simulink model "Torque_controller_using_LIM_wo_simulink"  (R2018a)
settings: Solver=VariableStepAuto  StartTime=0.0  StopTime=2  RelTol=1e-3
values from neighbouring files (symbols this model uses):
  fn = 100    [LIM_thrust_controller_parameters.m]    (also in lim_model_pu.m = 70)
  Ibase = Pn/(1.5*Vbase)    [LIM_thrust_controller_parameters.m]    (also in lim_model_pu.m)
  Imax = 4*Ibase    [LIM_thrust_controller_parameters.m]
  Imin = 0.1*Inom    (= 2.76073619632)    [LIM_thrust_controller_parameters.m]
  Inom = psi_ref/LM    (= 27.6073619632)    [LIM_thrust_controller_parameters.m]
  ki = ac^2*Lo    [LIM_thrust_controller_parameters.m]
  kp = ac*Lo    [LIM_thrust_controller_parameters.m]
  Lm = 32.6e-3    (= 0.0326)    [LIM_thrust_controller_parameters.m]    (also in lim_model.m; lim_model_pu.m = 32.6e-3/L_base)
  Lo = Ls    (= 0.0401)    [LIM_thrust_controller_parameters.m]
  Lr = 33.1e-3    (= 0.0331)    [LIM_thrust_controller_parameters.m]    (also in lim_model.m; lim_model_pu.m = 33.1e-3/L_base)
  p = 4    [LIM_thrust_controller_parameters.m]    (also in lim_model.m; lim_model_pu.m)
  Ra = ac*Lo - RR    [LIM_thrust_controller_parameters.m]
  RR = 2.7    [LIM_thrust_controller_parameters.m]
  tau = 0.2    [LIM_thrust_controller_parameters.m]    (also in lim_model.m = 0.066; lim_model_pu.m)
  Ts = 5e-6    (= 5e-06)    [LIM_thrust_controller_parameters.m]
  Tsc = 1/(fsw*50)    (= 1e-05)    [LIM_thrust_controller_parameters.m]
  Ty = Lr/RR    (= 0.0122592592593)    [LIM_thrust_controller_parameters.m]
  Vbase = Vn/sqrt(3)*sqrt(2)    [LIM_thrust_controller_parameters.m]    (also in lim_model_pu.m)
  w1 = 1    [LIM_thrust_controller_parameters.m]
  wbase = 2*pi*fn    (= 628.318530718)    [LIM_thrust_controller_parameters.m]    (also in lim_model_pu.m = 439.822971503)
  xi = (Lo+LM)/Lo    (= 1.81296758105)    [LIM_thrust_controller_parameters.m]
undefined symbols (not defined in the file or in its folder): DiscIntNeverNeededParam, id_ref, sigbuilder_block
libraries: powerlib_meascontrol x5, simulink x1
settings Model: Creator=akashsin  LastModifiedBy=akashsin

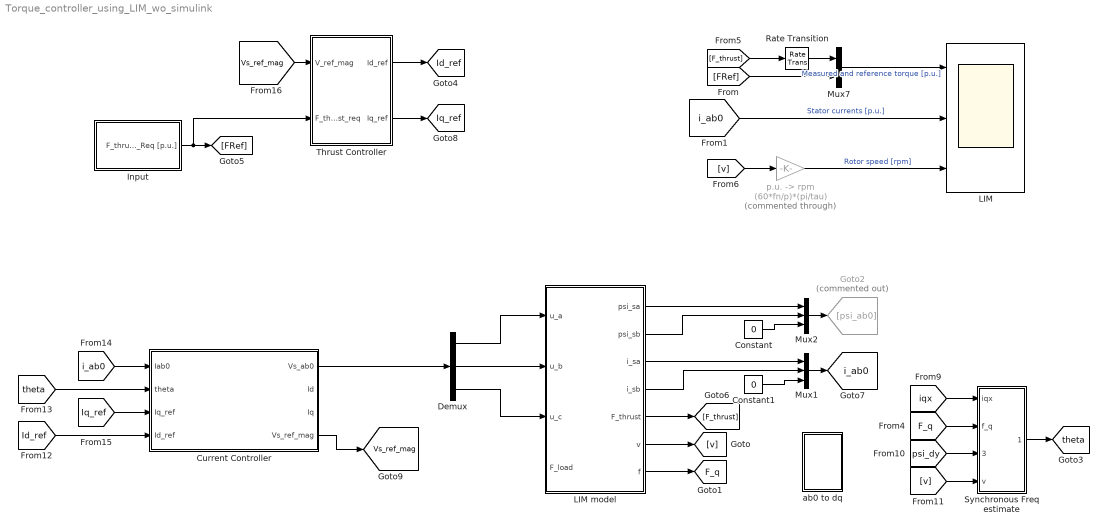
== system Torque_controller_using_LIM_wo_simulink ==
  Constant : Constant  Value=0  SampleTime=Tsc
  Constant1 : Constant  Value=0  SampleTime=Tsc
  Current Controller : Subsystem
  Demux : Demux  Outputs=3
  Goto2 : Goto  Commented=on  GotoTag=psi_ab0
  Input : Subsystem  Tag=STV Subsys  LoadFcn=sigbuilder_block('load');  StartFcn=sigbuilder_block('start');  StopFcn=sigbuilder_block('stop');  ClipboardFcn=sigbuilder_block('clipboard');  mask(Sigbuilder block){tuvar=[0:10]}
      mask help: Simulink:masks:SigbuilderBlock_MD
      mask init:
      | if ~strcmp(get_param(bdroot(gcbh),'SimulationStatus'),'stopped') tuvar = sigbuilder_block('maskInit'); end
      settings: CopyFcn=sigbuilder_block('copy');  DeleteFcn=sigbuilder_block('delete');  ModelCloseFcn=sigbuilder_block('modelClose');  PreSaveFcn=sigbuilder_block('preSave');  PauseFcn=sigbuilder_block('pause');  ContinueFcn=sigbuilder_block('continue');  NameChangeFcn=sigbuilder_block('namechange');  OpenFcn=sigbuilder_block('open',[683.25 241.5 615.75 445.5 ]);  CloseFcn=sigbuilder_block('close');
      mask Display: plot(0, 0, 100, 100,[2, 2, 32, 32, 2], [68, 8, 8, 68, 68],[32, 2], [38, 38], [32, 19, 2],[53, 60, 44], [32, 17, 17, 2],[16, 16, 31, 31]);txt = getActiveGroup(gcbh);text(2, 100, txt,'verticalAlignment', 'top');
  LIM : Scope  NumInputPorts=3
  LIM model : Subsystem
  Mux1 : Mux  Inputs=3
  Mux2 : Mux  Inputs=3
  Mux7 : Mux  Inputs=2
  Rate Transition : RateTransition  OutPortSampleTime=Tsc
  Synchronous Freq estimate : Subsystem
  Thrust Controller : Subsystem
  ab0 to dq : Subsystem
  "p.u. -> rpm" : Gain  Commented=through  Gain=(60*fn/p)*(pi/tau)
  tag scope: F_q=global, Id_ref=global, Iq_ref=global, Vs_ref_mag=global, i_ab0=global, theta=global
  wires:
  Thrust Controller/2(Iq_ref) -> [Iq_ref]
  Thrust Controller/1(Id_ref) -> [Id_ref]
  Input/1(F_thrust_Req [p.u.]) -> [FRef], Thrust Controller/2(F_thrust_req)
  [Vs_ref_mag] -> Thrust Controller/1(V_ref_mag)
  Synchronous Freq estimate/1(theta) -> [theta]
  [v] -> Synchronous Freq estimate/4(v)
  [psi_dy] -> Synchronous Freq estimate/3(psi_dy)
  [F_q] -> Synchronous Freq estimate/2(f_q)
  [iqx] -> Synchronous Freq estimate/1(iqx)
  Mux1/1 -> [i_ab0]
  LIM model/5(F_thrust) -> [F_thrust]
  Constant1/1 -> Mux1/3
  LIM model/4(i_sb) -> Mux1/2
  LIM model/3(i_sa) -> Mux1/1
  Mux2/1 -> Goto2/1
  Constant/1 -> Mux2/3
  LIM model/2(psi_sb) -> Mux2/2
  LIM model/1(psi_sa) -> Mux2/1
  LIM model/6(v) -> [v]
  LIM model/7(f) -> [F_q]
  Demux/3 -> LIM model/3(u_c)
  Demux/1 -> LIM model/1(u_a)
  Demux/2 -> LIM model/2(u_b)
  [FRef] -> Mux7/2
  [v] -> "p.u. -> rpm"/1
  "p.u. -> rpm"/1 -> LIM/3  "Rotor speed [rpm]"
  Mux7/1 -> LIM/1  "Measured and reference torque [p.u.]"
  Rate Transition/1 -> Mux7/1
  [F_thrust] -> Rate Transition/1
  [i_ab0] -> LIM/2  "Stator currents [p.u.]"
  Current Controller/4(Vs_ref_mag) -> [Vs_ref_mag]
  Current Controller/1(Vs_ab0) -> Demux/1
  [Id_ref] -> Current Controller/4(Id_ref)
  [Iq_ref] -> Current Controller/3(Iq_ref)
  [theta] -> Current Controller/2(theta)
  [i_ab0] -> Current Controller/1(Iab0)

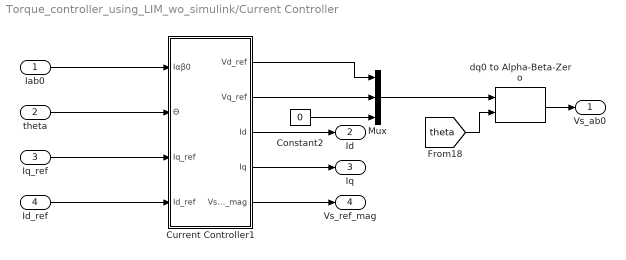
== system Torque_controller_using_LIM_wo_simulink/Current Controller ==
  Iab0 : Inport
  theta : Inport  Port=2
  Iq_ref : Inport  Port=3
  Id_ref : Inport  Port=4
  Constant2 : Constant  Value=0  SampleTime=Tsc
  Current Controller1 : Subsystem
  Mux : Mux  Inputs=3
  dq0 to Alpha-Beta-Zero : powerlib_meascontrol/Transformations/dq0 to Alpha-Beta-Zero  Alignment=Aligned with phase A axis
      settings: SourceProductName=Simscape Power Systems  SourceProductBaseCode=PS
  Vs_ab0 : Outport
  Id : Outport  Port=2
  Iq : Outport  Port=3
  Vs_ref_mag : Outport  Port=4
  wires:
  Current Controller1/5(Vs_ref_mag) -> Vs_ref_mag/1
  Id_ref/1 -> Current Controller1/4(Id_ref)
  Iab0/1 -> Current Controller1/1(Iαβ0)
  theta/1 -> Current Controller1/2(Θ)
  Iq_ref/1 -> Current Controller1/3(Iq_ref)
  Current Controller1/4(Iq) -> Iq/1
  [theta] -> dq0 to Alpha-Beta-Zero/2
  Mux/1 -> dq0 to Alpha-Beta-Zero/1
  dq0 to Alpha-Beta-Zero/1 -> Vs_ab0/1
  Current Controller1/3(Id) -> Id/1
  Constant2/1 -> Mux/3
  Current Controller1/2(Vq_ref) -> Mux/2
  Current Controller1/1(Vd_ref) -> Mux/1

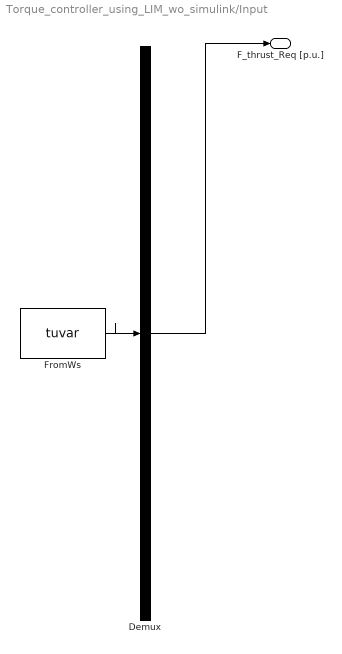
== system Torque_controller_using_LIM_wo_simulink/Input ==
  Demux : Demux  Tag=STV Demux  Outputs=1
  FromWs : FromWorkspace  Tag=STV FromWs  VariableName=tuvar  SampleTime=0
      SigBuilderData=|
      | common.afterFinalStr = 'Extrapolate'
      | common.sampleTime = 0
      | dataSet.timeRange = [0 2]
      | dataSet.name = 'Test 1'
      | sbobj.Groups.Name = 'Test 1'
      | sbobj.Groups.Signals.Name = 'F_thrust_Req [p.u.]'
      | sbobj.Groups.Signals.XData = [0 0.1 0.1 1.07 1.345 1.345 1.6 1.6 2]
      | sbobj.Groups.Signals.YData = [0 0 1.005 1.005 1.005 0.75 0.745 -0.005 -0.005]
      | sbobj.Groups.TimeRange = [0 2]
  F_thrust_Req [p.u.] : Outport  Tag=STV Outport
  wires:
  FromWs/1 -> Demux/1
  Demux/1 -> F_thrust_Req [p.u.]/1

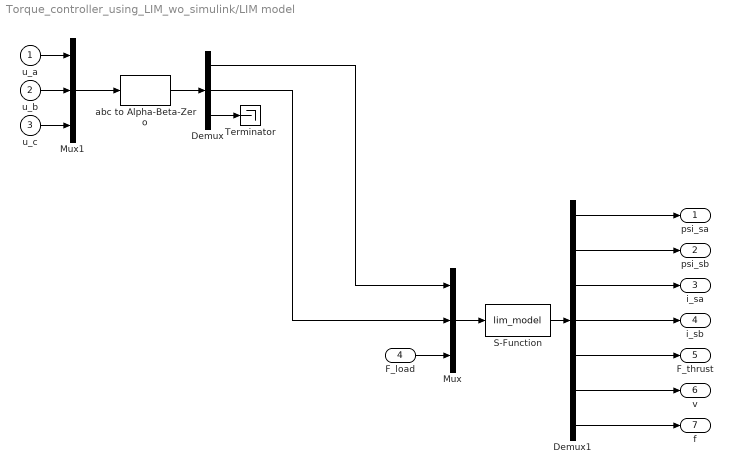
== system Torque_controller_using_LIM_wo_simulink/LIM model ==
  u_a : Inport
  u_b : Inport  Port=2
  u_c : Inport  Port=3
  F_load : Inport  Port=4
  Demux : Demux  Outputs=3
  Demux1 : Demux  Outputs=7
  Mux : Mux  Inputs=3
  Mux1 : Mux  Inputs=3
  S-Function : S-Function  FunctionName=lim_model  SFunctionDeploymentMode=off  EnableBusSupport=off
  Terminator : Terminator
  abc to Alpha-Beta-Zero : powerlib_meascontrol/Transformations/abc to Alpha-Beta-Zero
      settings: SourceProductName=Simscape Power Systems
  psi_sa : Outport
  psi_sb : Outport  Port=2
  i_sa : Outport  Port=3
  i_sb : Outport  Port=4
  F_thrust : Outport  Port=5
  v : Outport  Port=6
  f : Outport  Port=7
  wires:
  F_load/1 -> Mux/3
  Mux/1 -> S-Function/1
  Demux1/2 -> psi_sb/1
  Demux1/3 -> i_sa/1
  S-Function/1 -> Demux1/1
  Demux1/7 -> f/1
  Demux/1 -> Mux/1
  Demux1/4 -> i_sb/1
  Demux1/6 -> v/1
  Demux1/1 -> psi_sa/1
  Demux/2 -> Mux/2
  Demux1/5 -> F_thrust/1
  u_a/1 -> Mux1/1
  Demux/3 -> Terminator/1
  u_c/1 -> Mux1/3
  u_b/1 -> Mux1/2
  abc to Alpha-Beta-Zero/1 -> Demux/1
  Mux1/1 -> abc to Alpha-Beta-Zero/1

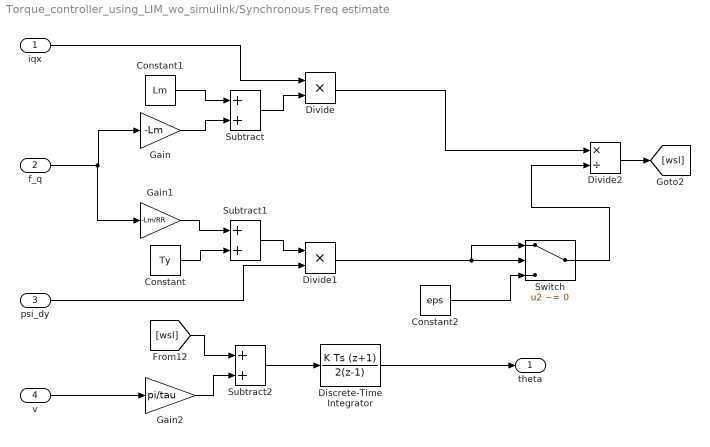
== system Torque_controller_using_LIM_wo_simulink/Synchronous Freq estimate ==
  iqx : Inport
  f_q : Inport  Port=2
  psi_dy : Inport  Port=3
  v : Inport  Port=4
  Constant : Constant  Value=Ty  SampleTime=Tsc
  Constant1 : Constant  Value=Lm  SampleTime=Tsc
  Constant2 : Constant  Value=eps  SampleTime=Tsc
  Discrete-Time Integrator : DiscreteIntegrator  IntegratorMethod=Integration: Trapezoidal  SampleTime=Tsc  ICPrevOutput=DiscIntNeverNeededParam  ICPrevScaledInput=DiscIntNeverNeededParam
  Divide : Product  Inputs=**
  Divide1 : Product  Inputs=**
  Divide2 : Product  Inputs=*/
  Gain : Gain  Gain=-Lm
  Gain1 : Gain  Gain=-Lm/RR
  Gain2 : Gain  Gain=pi/tau
  Subtract : Sum
  Subtract1 : Sum
  Subtract2 : Sum
  Switch : Switch  Criteria=u2 ~= 0
  theta : Outport
  wires:
  Divide2/1 -> [wsl]
  Switch/1 -> Divide2/2
  Constant2/1 -> Switch/3
  Divide1/1 -> Switch/2, Switch/1
  iqx/1 -> Divide/1
  v/1 -> Gain2/1
  Gain2/1 -> Subtract2/2
  Gain1/1 -> Subtract1/1
  Constant/1 -> Subtract1/2
  [wsl] -> Subtract2/1
  Divide/1 -> Divide2/1
  psi_dy/1 -> Divide1/2
  Subtract1/1 -> Divide1/1
  Gain/1 -> Subtract/2
  f_q/1 -> Gain/1, Gain1/1
  Discrete-Time Integrator/1 -> theta/1
  Subtract2/1 -> Discrete-Time Integrator/1
  Subtract/1 -> Divide/2
  Constant1/1 -> Subtract/1

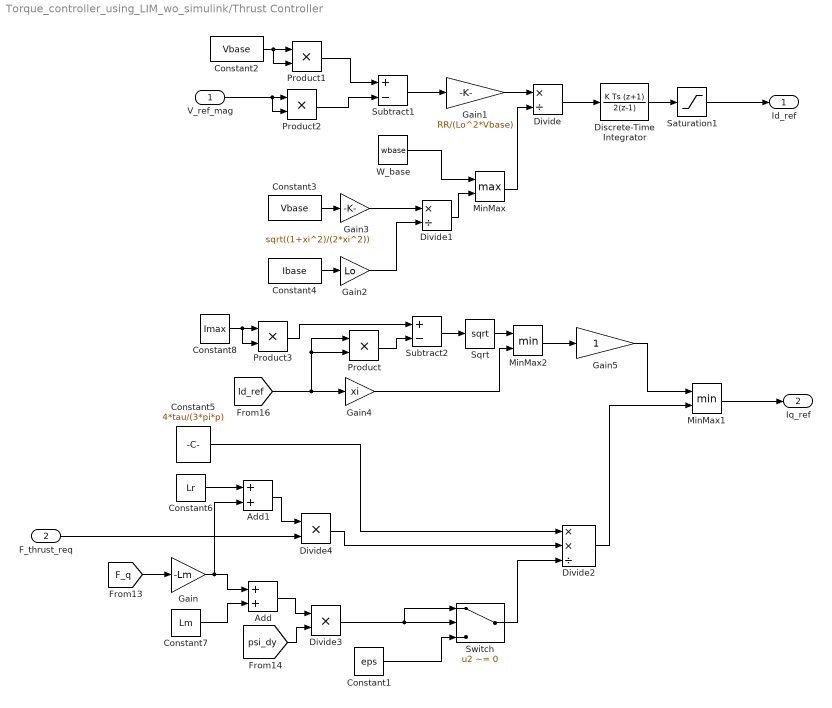
== system Torque_controller_using_LIM_wo_simulink/Thrust Controller ==
  V_ref_mag : Inport
  F_thrust_req : Inport  Port=2
  Add : Sum
  Add1 : Sum
  Constant1 : Constant  Value=eps  SampleTime=Tsc
  Constant2 : Constant  Value=Vbase  SampleTime=Tsc
  Constant3 : Constant  Value=Vbase  SampleTime=Tsc
  Constant4 : Constant  Value=Ibase  SampleTime=Tsc
  Constant5 : Constant  Value=4*tau/(3*pi*p)  SampleTime=Tsc
  Constant6 : Constant  Value=Lr  SampleTime=Tsc
  Constant7 : Constant  Value=Lm  SampleTime=Tsc
  Constant8 : Constant  Value=Imax  SampleTime=Tsc
  Discrete-Time Integrator : DiscreteIntegrator  IntegratorMethod=Integration: Trapezoidal  SampleTime=Ts  ICPrevOutput=DiscIntNeverNeededParam  ICPrevScaledInput=DiscIntNeverNeededParam
  Divide : Product  Inputs=*/
  Divide1 : Product  Inputs=*/
  Divide2 : Product  Inputs=**/
  Divide3 : Product  Inputs=**
  Divide4 : Product  Inputs=**
  Gain : Gain  Gain=-Lm
  Gain1 : Gain  Gain=RR/(Lo^2*Vbase)
  Gain2 : Gain  Gain=Lo
  Gain3 : Gain  Gain=sqrt((1+xi^2)/(2*xi^2))
  Gain4 : Gain  Gain=xi
  Gain5 : Gain
  MinMax : MinMax  Function=max  Inputs=2
  MinMax1 : MinMax  Inputs=2
  MinMax2 : MinMax  Inputs=2
  Product{,1..3} (4 alike) : Product
  Saturation1 : Saturate  UpperLimit=Inom  LowerLimit=Imin
  Sqrt : Sqrt  SaturateOnIntegerOverflow=on
  Subtract1 : Sum  Inputs=+-
  Subtract2 : Sum  Inputs=+-
  Switch : Switch  Criteria=u2 ~= 0
  W_base : Constant  Value=wbase  SampleTime=Tsc
  Id_ref : Outport
  Iq_ref : Outport  Port=2
  wires:
  Switch/1 -> Divide2/3
  Constant1/1 -> Switch/3
  Divide3/1 -> Switch/2, Switch/1
  Gain2/1 -> Divide1/2
  Product1/1 -> Subtract1/1
  Constant3/1 -> Gain3/1
  Gain5/1 -> MinMax1/1
  Gain1/1 -> Divide/1
  Subtract1/1 -> Gain1/1
  MinMax2/1 -> Gain5/1
  V_ref_mag/1 -> Product2/1, Product2/2
  Subtract2/1 -> Sqrt/1
  Product3/1 -> Subtract2/1
  Divide1/1 -> MinMax/2
  Gain4/1 -> MinMax2/2
  MinMax1/1 -> Iq_ref/1
  Constant4/1 -> Gain2/1
  Sqrt/1 -> MinMax2/1
  Product/1 -> Subtract2/2
  Constant8/1 -> Product3/1, Product3/2
  Constant5/1 -> Divide2/1
  Divide/1 -> Discrete-Time Integrator/1
  MinMax/1 -> Divide/2
  Discrete-Time Integrator/1 -> Saturation1/1
  Product2/1 -> Subtract1/2
  Constant6/1 -> Add1/1
  [Id_ref] -> Gain4/1, Product/1, Product/2
  [psi_dy] -> Divide3/2
  Divide2/1 -> MinMax1/2
  Add/1 -> Divide3/1
  Add1/1 -> Divide4/1
  [F_q] -> Gain/1
  W_base/1 -> MinMax/1
  Saturation1/1 -> Id_ref/1
  Constant7/1 -> Add/2
  Constant2/1 -> Product1/1, Product1/2
  Gain3/1 -> Divide1/1
  Divide4/1 -> Divide2/2
  Gain/1 -> Add/1, Add1/2
  F_thrust_req/1 -> Divide4/2

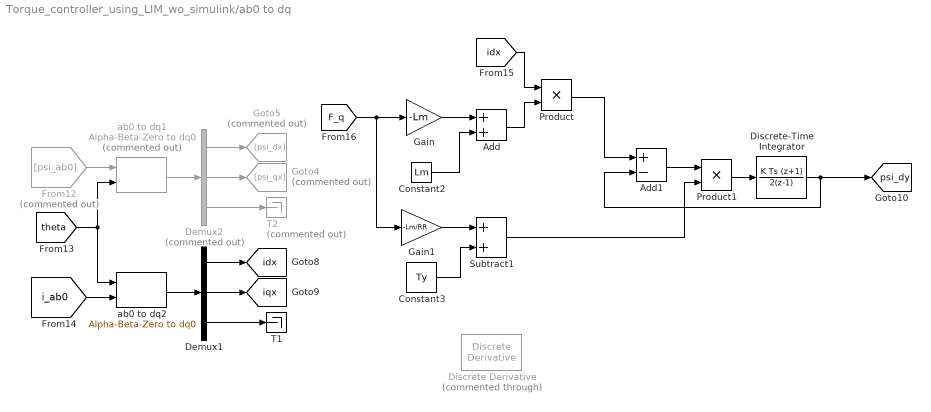
== system Torque_controller_using_LIM_wo_simulink/ab0 to dq ==
  Add : Sum
  Add1 : Sum  Inputs=+-
  Constant2 : Constant  Value=Lm  SampleTime=Tsc
  Constant3 : Constant  Value=Ty  SampleTime=Tsc
  Demux1 : Demux  Outputs=3
  Demux2 : Demux  Commented=on  Outputs=3
  Discrete Derivative : simulink/Quick Insert/Discrete/Discrete Derivative  Commented=through  gainval=1.0  ICPrevScaledInput=0.0  OutMin=[]  OutMax=[]  OutDataType=fixdt(1, 16)  OutScaling=2^-10  DoSatur=off
      settings: SourceProductName=Simulink  SourceProductBaseCode=SL
  Discrete-Time Integrator : DiscreteIntegrator  IntegratorMethod=Integration: Trapezoidal  SampleTime=Tsc  ICPrevOutput=DiscIntNeverNeededParam  ICPrevScaledInput=DiscIntNeverNeededParam
  From12 : From  Commented=on  GotoTag=psi_ab0
  Gain : Gain  Gain=-Lm
  Gain1 : Gain  Gain=-Lm/RR
  Goto4 : Goto  Commented=on  GotoTag=psi_qx
  Goto5 : Goto  Commented=on  GotoTag=psi_dx
  Product : Product
  Product1 : Product
  Subtract1 : Sum
  T1 : Terminator
  T2 : Terminator  Commented=on
  ab0 to dq1 : powerlib_meascontrol/Transformations/Alpha-Beta-Zero to dq0  Commented=on  Alignment=Aligned with phase A axis
      settings: SourceProductName=Simscape Power Systems
  ab0 to dq2 : powerlib_meascontrol/Transformations/Alpha-Beta-Zero to dq0  Alignment=Aligned with phase A axis
      settings: SourceProductName=Simscape Power Systems
  tag scope: idx=global, iqx=global, psi_dy=global
  wires:
  Add/1 -> Product/2
  Discrete-Time Integrator/1 -> Add1/2, [psi_dy]
  Product1/1 -> Discrete-Time Integrator/1
  Subtract1/1 -> Product1/2
  Add1/1 -> Product1/1
  Demux1/1 -> [idx]
  Gain1/1 -> Subtract1/1
  Product/1 -> Add1/1
  [i_ab0] -> ab0 to dq2/1
  Constant2/1 -> Add/2
  Demux2/1 -> Goto5/1
  ab0 to dq1/1 -> Demux2/1
  Demux2/2 -> Goto4/1
  From12/1 -> ab0 to dq1/1
  Demux1/2 -> [iqx]
  Gain/1 -> Add/1
  Demux1/3 -> T1/1
  ab0 to dq2/1 -> Demux1/1
  [idx] -> Product/1
  Demux2/3 -> T2/1
  Constant3/1 -> Subtract1/2
  [theta] -> ab0 to dq1/2, ab0 to dq2/2
  [F_q] -> Gain/1, Gain1/1

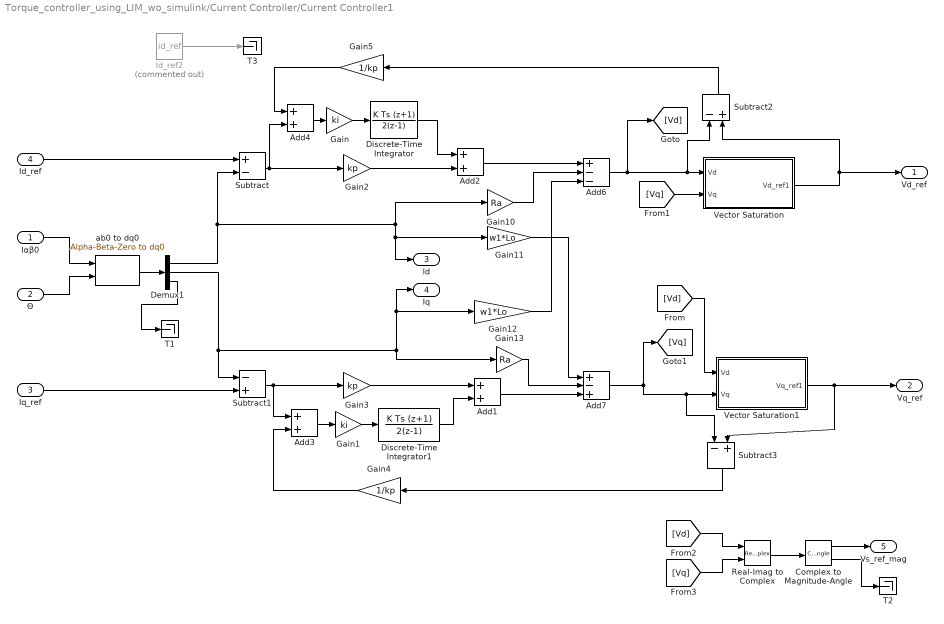
== system Torque_controller_using_LIM_wo_simulink/Current Controller/Current Controller1 ==
  Iαβ0 : Inport
  Θ : Inport  Port=2
  Iq_ref : Inport  Port=3
  Id_ref : Inport  Port=4
  Add{1..4} (4 alike) : Sum
  Add6 : Sum  Inputs=+--
  Add7 : Sum  Inputs=+-+
  Complex to Magnitude-Angle : ComplexToMagnitudeAngle
  Demux1 : Demux  Outputs=3
  Discrete-Time Integrator : DiscreteIntegrator  IntegratorMethod=Integration: Trapezoidal  SampleTime=Ts  ICPrevOutput=DiscIntNeverNeededParam  ICPrevScaledInput=DiscIntNeverNeededParam
  Discrete-Time Integrator1 : DiscreteIntegrator  IntegratorMethod=Integration: Trapezoidal  SampleTime=Ts  ICPrevOutput=DiscIntNeverNeededParam  ICPrevScaledInput=DiscIntNeverNeededParam
  Gain : Gain  Gain=ki
  Gain1 : Gain  Gain=ki
  Gain10 : Gain  Gain=Ra
  Gain11 : Gain  Gain=w1*Lo
  Gain12 : Gain  Gain=w1*Lo
  Gain13 : Gain  Gain=Ra
  Gain2 : Gain  Gain=kp
  Gain3 : Gain  Gain=kp
  Gain4 : Gain  Gain=1/kp
  Gain5 : Gain  Gain=1/kp
  Id_ref2 : Constant  Commented=on  Value=id_ref
  Real-Imag to Complex : RealImagToComplex
  Subtract : Sum  Inputs=+-
  Subtract1 : Sum  Inputs=-+
  Subtract2 : Sum  Inputs=-+
  Subtract3 : Sum  Inputs=-+
  T1 : Terminator
  T2 : Terminator
  T3 : Terminator
  Vector Saturation : Subsystem
  Vector Saturation1 : Subsystem
  ab0 to dq0 : powerlib_meascontrol/Transformations/Alpha-Beta-Zero to dq0  Alignment=Aligned with phase A axis
      settings: SourceProductName=Simscape Power Systems
  Vd_ref : Outport
  Vq_ref : Outport  Port=2
  Id : Outport  Port=3
  Iq : Outport  Port=4
  Vs_ref_mag : Outport  Port=5
  wires:
  Id_ref/1 -> Subtract/1
  [Vq] -> Real-Imag to Complex/2
  [Vd] -> Real-Imag to Complex/1
  Id_ref2/1 -> T3/1
  Complex to Magnitude-Angle/2 -> T2/1
  Complex to Magnitude-Angle/1 -> Vs_ref_mag/1
  Real-Imag to Complex/1 -> Complex to Magnitude-Angle/1
  Vector Saturation/1(Vd_ref1) -> Subtract2/2, Vd_ref/1
  Vector Saturation1/1(Vq_ref1) -> Subtract3/2, Vq_ref/1
  [Vq] -> Vector Saturation/2(Vq)
  [Vd] -> Vector Saturation1/1(Vd)
  Θ/1 -> ab0 to dq0/2
  Add7/1 -> [Vq], Vector Saturation1/2(Vq), Subtract3/1
  Add6/1 -> [Vd], Vector Saturation/1(Vd), Subtract2/1
  Iq_ref/1 -> Subtract1/2
  Gain13/1 -> Add7/2
  Gain12/1 -> Add6/3
  Demux1/2 -> Subtract1/1, Gain13/1, Iq/1, Gain12/1
  Add1/1 -> Add7/3
  Add2/1 -> Add6/1
  Gain11/1 -> Add7/1
  Gain10/1 -> Add6/2
  Demux1/1 -> Subtract/2, Gain10/1, Id/1, Gain11/1
  Subtract2/1 -> Gain5/1
  Add4/1 -> Gain/1
  Subtract1/1 -> Gain3/1, Add3/1
  Gain1/1 -> Discrete-Time Integrator1/1
  Gain/1 -> Discrete-Time Integrator/1
  Subtract/1 -> Gain2/1, Add4/2
  ab0 to dq0/1 -> Demux1/1
  Demux1/3 -> T1/1
  Iαβ0/1 -> ab0 to dq0/1
  Gain5/1 -> Add4/1
  Gain2/1 -> Add2/2
  Gain4/1 -> Add3/2
  Add3/1 -> Gain1/1
  Discrete-Time Integrator/1 -> Add2/1
  Subtract3/1 -> Gain4/1
  Discrete-Time Integrator1/1 -> Add1/2
  Gain3/1 -> Add1/1

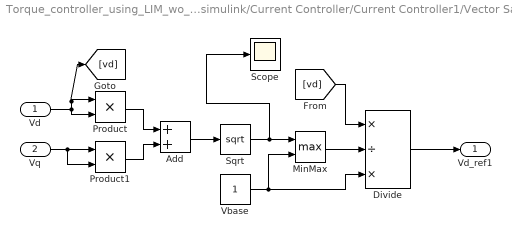
== system Torque_controller_using_LIM_wo_simulink/Current Controller/Current Controller1/Vector Saturation ==
  Vd : Inport
  Vq : Inport  Port=2
  Add : Sum
  Divide : Product  Inputs=*/*
  MinMax : MinMax  Function=max  Inputs=2
  Product : Product
  Product1 : Product
  Scope : Scope
  Sqrt : Sqrt  SaturateOnIntegerOverflow=on
  Vbase : Constant
  Vd_ref1 : Outport
  wires:
  Vbase/1 -> MinMax/2, Divide/3
  MinMax/1 -> Divide/2
  Vd/1 -> Product/2, Product/1, [vd]
  Product/1 -> Add/1
  Vq/1 -> Product1/1, Product1/2
  Product1/1 -> Add/2
  Add/1 -> Sqrt/1
  Sqrt/1 -> MinMax/1, Scope/1
  [vd] -> Divide/1
  Divide/1 -> Vd_ref1/1

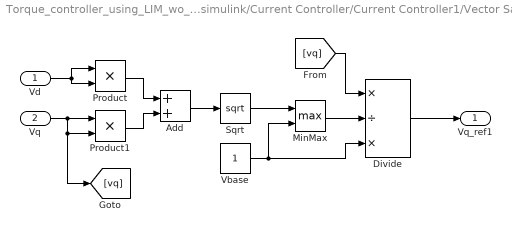
== system Torque_controller_using_LIM_wo_simulink/Current Controller/Current Controller1/Vector Saturation1 ==
  Vd : Inport
  Vq : Inport  Port=2
  Add : Sum
  Divide : Product  Inputs=*/*
  MinMax : MinMax  Function=max  Inputs=2
  Product : Product
  Product1 : Product
  Sqrt : Sqrt  SaturateOnIntegerOverflow=on
  Vbase : Constant
  Vq_ref1 : Outport
  wires:
  Vbase/1 -> MinMax/2, Divide/3
  MinMax/1 -> Divide/2
  Vd/1 -> Product/2, Product/1
  Product/1 -> Add/1
  Vq/1 -> Product1/1, Product1/2, [vq]
  Product1/1 -> Add/2
  Add/1 -> Sqrt/1
  Sqrt/1 -> MinMax/1
  [vq] -> Divide/1
  Divide/1 -> Vq_ref1/1
